simulink model "BattEv"  (R2024a)
settings: Solver=VariableStepAuto  StartTime=0.0  StopTime=inf  RelTol=1e-3  EnableMultiTasking=on
model workspace (MAT data in the model file):
  BattCapInit = Simulink.Parameter
  BattCapInit.Value = 3.6
  BattCapInit.Complexity = 'real'
  BattCapInit.Dimensions = [1 1]
  BattCapInit.DataType = 'double'
  BattChargeMax = Simulink.Parameter
  BattChargeMax.Value = 4.8
  BattChargeMax.Complexity = 'real'
  BattChargeMax.Dimensions = [1 1]
  BattChargeMax.DataType = 'double'
  BattTempBp = Simulink.Parameter
  BattTempBp.Value = [263.15 273.15 298.15 313.15]
  BattTempBp.Complexity = 'real'
  BattTempBp.Dimensions = [1 4]
  BattTempBp.DataType = 'double'
  CapLUTBp = Simulink.Parameter
  CapLUTBp.Value = [0.01 0.02 0.03 0.04 0.05 0.06 0.07 0.08 0.09 0.1 0.11 0.12 0.13 0.14 0.15 0.16 0.17 0.18 0.19 0.2 0.21 0.22 0.23 0.24 0.25 0.26 0.27 0.28 0.29 0.3 0.31 0.32 0.33 0.34 0.35 0.36 0.37 0.38 0.39 0.4 0.41 0.42 0.43 0.44 0.45 0.46 0.47 0.48 0.49 0.5 0.51 0.52 0.53 0.54 0.55 0.56 0.57 0.58 0.59 0.6 0.61 0.62 0.63 0.64 0.65 0.66 0.67 0.68 0.69 0.7 0.71 0.72 0.73 0.74 0.75 0.76 0.77 0.78 0.79 0.8 0.81 0.82 0.83 0.84 0.85 0.86 0.87 0.88 0.89 0.9 0.91 0.92 0.93 0.94 0.95 0.96 0.97 0.98 0.99 1]
  CapLUTBp.Complexity = 'real'
  CapLUTBp.Dimensions = [1 100]
  CapLUTBp.DataType = 'double'
  CapSOCBp = Simulink.Parameter
  CapSOCBp.Value = [0.01 0.02 0.03 0.04 0.05 0.06 0.07 0.08 0.09 0.1 0.11 0.12 0.13 0.14 0.15 0.16 0.17 0.18 0.19 0.2 0.21 0.22 0.23 0.24 0.25 0.26 0.27 0.28 0.29 0.3 0.31 0.32 0.33 0.34 0.35 0.36 0.37 0.38 0.39 0.4 0.41 0.42 0.43 0.44 0.45 0.46 0.47 0.48 0.49 0.5 0.51 0.52 0.53 0.54 0.55 0.56 0.57 0.58 0.59 0.6 0.61 0.62 0.63 0.64 0.65 0.66 0.67 0.68 0.69 0.7 0.71 0.72 0.73 0.74 0.75 0.76 0.77 0.78 0.79 0.8 0.81 0.82 0.83 0.84 0.85 0.86 0.87 0.88 0.89 0.9 0.91 0.92 0.93 0.94 0.95 0.96 0.97 0.98 0.99 1]
  CapSOCBp.Complexity = 'real'
  CapSOCBp.Dimensions = [1 100]
  CapSOCBp.DataType = 'double'
  Em = Simulink.Parameter
  Em.Value = [3.01162183959; 3.0857565027; 3.14177499163; 3.18631823552; 3.22334954768; 3.25390136234; 3.27878869705; 3.30070350874; 3.32118523631; 3.33873222863; 3.35681278765; 3.37271031815; 3.38793252475; 3.40246133853; 3.41323877472; 3.42274053961; 3.43230513034; 3.4412706664; 3.45046092538; 3.46050021597; 3.47059444209; 3.47754582202; 3.48403887677; 3.49083263176; 3.49762638675; 3.50414427849; 3.51006189737; 3.51650779121; 3.52300031606; 3.5294928409; 3.53574150484; 3.54126505717; 3.54599126111; 3.55084210438; 3.55569196095; 3.56052372392; 3.56532059653; 3.56979945432; 3.57444121268; 3.57904303347; 3.58364485425; 3.58840361875; 3.59316763087; 3.59914045642; 3.60536834334; 3.61166009905; 3.61797346412; 3.6242868292; 3.63060019428; 3.63762035332; 3.64493091714; 3.65193784155; 3.65894476597; 3.66595169039; 3.67346631196; 3.68205597287; 3.69093403907; 3.69981210527; 3.70876940775; 3.71776352137; 3.72686785651; 3.73538877817; 3.7438965512; 3.75240319274; 3.76046489817; 3.76888762107; 3.7779024494; 3.78684332393; 3.79578419847; 3.80453642297; 3.81235798589; 3.82032795055; 3.82829600796; 3.83626406537; 3.84436267546; 3.85250733117; 3.86057855537; 3.86864977957; 3.87672100377; 3.88493610528; 3.89310639829; 3.90173837212; 3.91095173578; 3.92144530461; 3.93240377768; 3.94373568414; 3.95558619351; 3.96743304428; 3.97920029575; 3.99089798499; 4.00334195303; 4.01527114968; 4.02728436042; 4.039094143; 4.04916289178; 4.05870791988; 4.06775178123; 4.07651000375; 4.08674414955; 4.1040722857]
  Em.Complexity = 'real'
  Em.Dimensions = [100 1]
  Em.DataType = 'double'
  Np = Simulink.Parameter
  Np.Value = 31
  Np.Complexity = 'real'
  Np.Dimensions = [1 1]
  Np.DataType = 'double'
  Ns = Simulink.Parameter
  Ns.Value = 96
  Ns.Complexity = 'real'
  Ns.Dimensions = [1 1]
  Ns.DataType = 'double'
  RInt = Simulink.Parameter
  RInt.Value = [0.0569026752707 0.0629164241673 0.108383589577 0.108526908513 0.0575506938969 0.0627185254642 0.104276452251 0.117675091219 0.0576730924021 0.0627490000658 0.0975073630061 0.123235721151 ... (400 elements, 4x100)]
  RInt.Complexity = 'real'
  RInt.Dimensions = [4 100]
  RInt.DataType = 'double'
undefined symbols (not defined in the file): BattSocInit
libraries: autolibdatasheetbattery x1
settings Model: DataDictionary=BMS_Software_DD.sldd  ModifiedByFormat=The MathWorks, Inc.  SimulationMode=accelerator  PauseTimes=10  Creator=The MathWorks, Inc.  LastModifiedBy=The MathWorks, Inc.
settings SolverCC: AlgebraicLoopSolver=TrustRegion  MaxZcPerStep=1
settings DataIOCC: DSMLogging=off  ReturnWorkspaceOutputs=off
settings OptimizationCC: ReuseModelBlockBuffer=off
settings DebuggingCC: UnderspecifiedInitializationDetection=Classic  MergeDetectMultiDrivingBlocksExec=none  UnconnectedInputMsg=warning  UnconnectedOutputMsg=warning  UnconnectedLineMsg=warning  SubsystemReferenceDiagnosticForUnitTest=warning  ArithmeticOperatorsInVariantConditions=warning
settings ModelReferenceCC: EnableRefExpFcnMdlSchedulingChecks=on  PropagateSignalLabelsOutOfModel=off
settings SFSimCC: SimUseLocalCustomCode=off  CustomCodeUndefinedFunction=UseInterfaceOnly
settings RTWCC: RTWUseLocalCustomCode=off  GPUComputeCapability=3.5  DLArmComputeVersion=19.05
settings CodeAppCC: StateflowObjectComments=on
settings GRTTargetCC: TargetLangStandard=C89/C90 (ANSI)
settings ConfigComp: CovMetricSettings=dsw  CovSaveCumulativeToWorkspaceVar=on  CovSaveSingleToWorkspaceVar=on  CovExternalEMLEnable=off
settings SimscapeCC: SimscapeNormalizeSystem=off

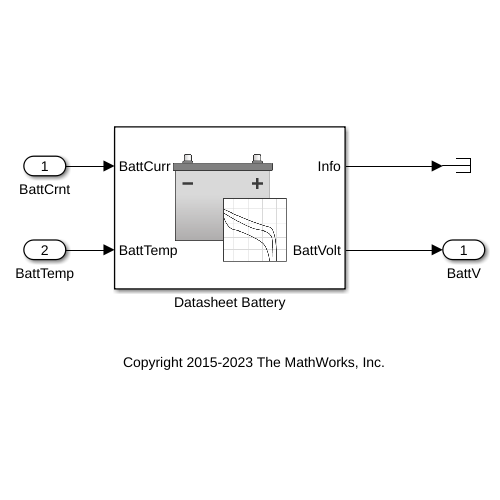
[thumbnail: Simulink's stored preview of the top-level diagram]
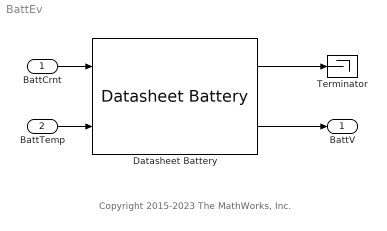
== system BattEv ==
  note: Copyright 2015-2023 The MathWorks, Inc.
  BattCrnt : Inport
  BattTemp : Inport  Port=2
  Datasheet Battery : autolibdatasheetbattery/Datasheet Battery  CapacityCtrl=Parameter  OutputVlt=Unfiltered  BattChargeMax=BattChargeMax  Em=Em*1  CapLUTBp=CapLUTBp  RInt=RInt  BattTempBp=BattTempBp  CapSOCBp=CapSOCBp  Ns=Ns  Np=Np  BattCapInit=BattSocInit*BattChargeMax  Tc=1/1000  Vinit=4.221  RefBlkName='autolibdatasheetbattery/Datasheet Battery'
  Terminator : Terminator
  BattV : Outport  VectorParamsAs1DForOutWhenUnconnected=off
  wires:
  Datasheet Battery/2 -> BattV/1
  BattTemp/1 -> Datasheet Battery/2
  BattCrnt/1 -> Datasheet Battery/1
  Datasheet Battery/1 -> Terminator/1
